simulink model "Controller"  (R2015a)
settings: Solver=ode3  SolverMode=SingleTasking  StartTime=0.0  StopTime=100  FixedStep=T_sim  RelTol=1e-3
PreLoadFcn:
  | LoadLibraries
values from neighbouring files (symbols this model uses):
  a = 10.26    [SetupComplete.m]
  A_x = 0.015    [SetupComplete.m]
  A_y = A_x    (= 0.015)    [SetupComplete.m]
  A_z = 0.16    [SetupComplete.m]
  C_d0 = 0.001193    [SetupComplete.m]
  C_x = 1.2    [SetupComplete.m]
  C_y = C_x    (= 1.2)    [SetupComplete.m]
  C_z = 2.2    [SetupComplete.m]
  CG_0 = [0,0,0.02]'    [SetupComplete.m]
  eta_23 = deg2rad(-1.42)    [Run3Copter.m]
  g = 9.81    [SetupComplete.m]
  h = 0.08    [SetupComplete.m]
  h_M = 0.064    [SetupComplete.m]
  I_BAC_0 = [ Ix,0,Ixz;0,Iy,0;Ixz,0,Iz]    [SetupComplete.m]
  Initial_Omegas = [1;1;1]*Omega_hover    [Run3Copter.m]
  l = 0.3450    (= 0.345)    [NDI_components.m]    (also in SetupComplete.m; robust_controller.m)
  l_arm = 0.264    [SetupComplete.m]
  m = 3.51    [SetupComplete.m]
  m_0 = 2.61    [SetupComplete.m]
  m_M = 0.300    (= 0.3)    [SetupComplete.m]
  R = 0.1778    [SetupComplete.m]    (also in robust_controller.m = eye(4))
  rho = 1.15    [SetupComplete.m]
  sigma = b*c/(pi*R)    (= 0.107416159567)    [SetupComplete.m]
  theta_0 = 0.38397    [SetupComplete.m]
  theta_1 = -0.2967    [SetupComplete.m]
  v_i0 = sqrt( 1/3*m*g/(2*rho*pi*R^2)  )    [SetupComplete.m]
undefined symbols (not defined in the file or in its folder): DOWN_0, EAST_0, Motor, NORTH_0, P_0, Prop, Q_0, R_0, Throttle_Hover, U_0, V_0, v_i_adim, Vx_adim, Vz_adim, W_0
undefined symbols (not defined in the file): Initial_Torques, J_FA, J_T, Rotation_sign, Tau_motors
libraries: XXCopter x39, simulink x35, vrlib x15, simulink_extras x7, aerolib6dofsys x2, qcatlib x2, dspinverses x2
(part 1 of 10)
settings Model: ExtModeTrigDuration=5000  Creator=DavidTorres  LastModifiedBy=juan
settings OptimizationCC: BlockReduction=off  BooleanDataType=off
settings DebuggingCC: SaveWithParameterizedLinksMsg=none  UnderspecifiedInitializationDetection=Classic  MergeDetectMultiDrivingBlocksExec=none
settings HardwareCC: TargetUnknown=on

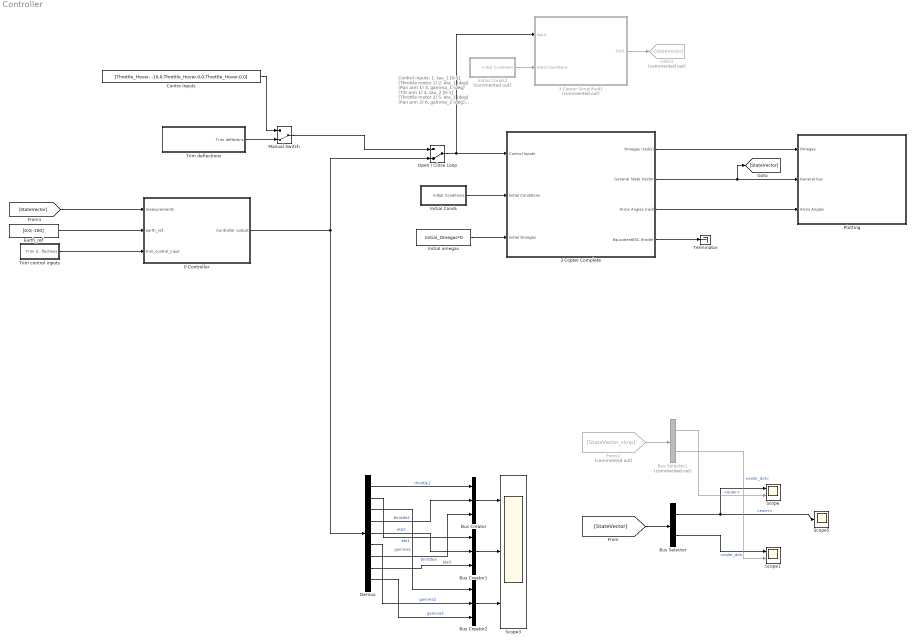
== system Controller ==
  note: Control inputs:
      | 1. tau_1 [0-1] (Throttle motor 1)
      | 2. eta_1 (deg)  (Pan arm 1)
      | 3. gamma_1 (deg)  (Tilt arm 1)
      |
      | 4. tau_2 [0-1] (Throttle motor 2)
      | 5. eta_2 (deg)  (Pan arm 2)
      | 6. gamma_2 (deg)  (Tilt arm 2)
      |
      | 7. tau_3 [0-1] (Throttle motor 3)
      | 8. eta_3 (deg)  (Pan arm  3)
      | 9. gamma_3 (deg)  (Tilt arm 3)
  3 Copter Complete : Subsystem
  3 Copter Simplified1 : Subsystem  Commented=on
  Bus Creator : BusCreator  Inputs=3
  Bus Creator1 : BusCreator  Inputs=3
  Bus Creator2 : BusCreator  Inputs=3
  Bus Selector : BusSelector  OutputSignals=euler,euler_dot
  Bus Selector1 : BusSelector  Commented=on  OutputSignals=euler,euler_dot
  Contro Inputs : Constant  Value=[Throttle_Hover, -10,0,Throttle_Hover,0,0,Throttle_Hover,0,0]
  Demux : Demux  Outputs=9
  Earth_ref : Constant  Value=[0;0;-100]
  From2 : From  Commented=on  GotoTag=StateVector_simp
  Goto1 : Goto  Commented=on  GotoTag=StateVector
  Initial Conds : Subsystem  TreatAsAtomicUnit=on
  Initial Conds2 : Subsystem  Commented=on  TreatAsAtomicUnit=on
  Initial omegas : Constant  Value=Initial_Omegas*0
  Manual Switch : ManualSwitch  CurrentSetting=0
  Open / Close Loop : ManualSwitch  CurrentSetting=0
  P Controller : Subsystem  Variant=on  OverrideUsingVariant=Variant1
  Plotting : Subsystem
  Scope : Scope  NumInputPorts=2
      settings: YMin=-0.5~-1  YMax=0.5~1  SaveName=ScopeData3
  Scope1 : Scope  NumInputPorts=2
      settings: YMin=-5~-5  YMax=5~5  SaveName=ScopeData4
  Scope3 : Scope  NumInputPorts=3
      settings: ShowLegends=on  TimeRange=100  YMin=0~-6~-1  YMax=1~1~1  SaveName=ScopeData6
  Scope5 : Scope
      settings: YMin=-0.002  YMax=0.01  SaveName=ScopeData13
  Terminator : Terminator
  Trim control inputs : Subsystem  TreatAsAtomicUnit=on
  Trim deflections : Subsystem  TreatAsAtomicUnit=on
  wires:
  Initial omegas/1 -> 3 Copter Complete/3(Initial Omegas)
  Initial Conds/1(Initial Conditions) -> 3 Copter Complete/2(Initial Conditions)
  3 Copter Complete/1(Omegas (rad/s)) -> Plotting/1(Omegas)
  3 Copter Complete/3(Arms Angles (rad)) -> Plotting/3(Arms Angles)
  Contro Inputs/1 -> Manual Switch/1
  Trim deflections/1(Trim deflectins) -> Manual Switch/2
  3 Copter Complete/2(General State Vector) -> [StateVector], Plotting/2(General bus)
  Manual Switch/1 -> Open / Close Loop/1
  [StateVector] -> P Controller/1(measurements)
  P Controller/1(Controller output) -> Demux/1, Open / Close Loop/2
  Trim control inputs/1(Trim deflections) -> P Controller/3(trim_control_input)
  Bus Selector/2 -> Scope1/1  "<euler_dot>"
  Bus Selector/1 -> Scope5/1, Scope/1  "<euler>"
  [StateVector] -> Bus Selector/1
  Demux/2 -> Bus Creator1/1  "eta1"
  Bus Creator/1 -> Scope3/1
  Demux/1 -> Bus Creator/1  "throttle1"
  Demux/4 -> Bus Creator/2  "throttle2"
  Demux/7 -> Bus Creator/3  "throttle3"
  Earth_ref/1 -> P Controller/2(earth_ref)
  3 Copter Complete/4(EquivalentESC throtle) -> Terminator/1
  Initial Conds2/1(Initial Conditions) -> 3 Copter Simplified1/2(Initial Conditions)
  3 Copter Simplified1/1(Out1) -> Goto1/1
  Open / Close Loop/1 -> 3 Copter Complete/1(Control Inputs), 3 Copter Simplified1/1(Input)
  Bus Selector1/2 -> Scope1/2  "<euler_dot>"
  Bus Selector1/1 -> Scope/2  "<euler>"
  From2/1 -> Bus Selector1/1
  Bus Creator1/1 -> Scope3/2
  Demux/5 -> Bus Creator1/2  "eta2"
  Demux/8 -> Bus Creator1/3  "eta3"
  Bus Creator2/1 -> Scope3/3
  Demux/3 -> Bus Creator2/1  "gamma1"
  Demux/6 -> Bus Creator2/2  "gamma2"
  Demux/9 -> Bus Creator2/3  "gamma3"

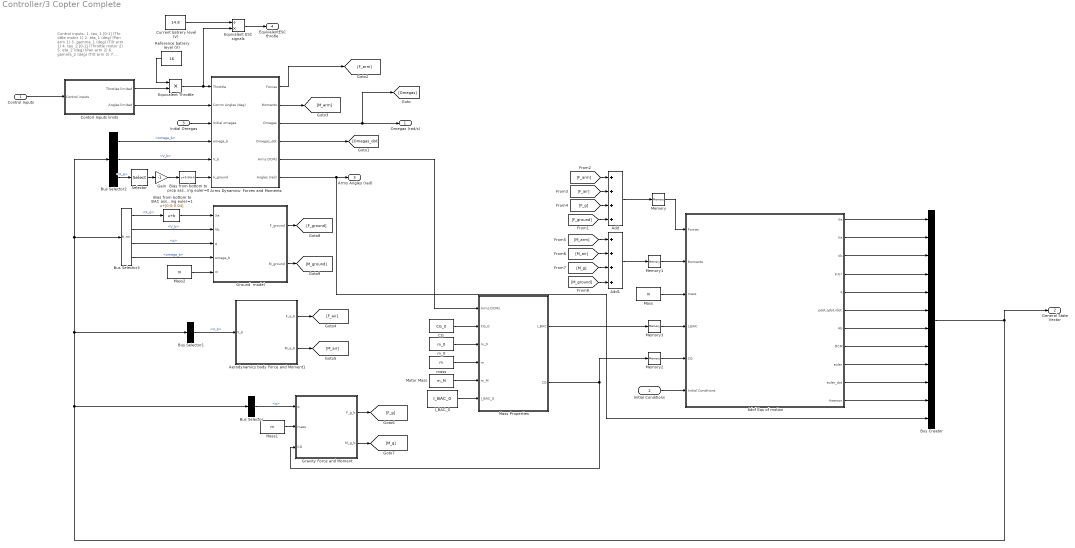
== system Controller/3 Copter Complete ==
  note: Control inputs:
      | 1. tau_1 [0-1] (Thr ottle motor 1)
      | 2. eta_1 (deg)  (Pan arm 1)
      | 3. gamma_1 (deg)  (Tilt arm 1)
      |
      | 4. tau_2 [0-1] (Throttle motor 2)
      | 5. eta_2 (deg)  (Pan arm 2)
      | 6. gamma_2 (deg)  (Tilt arm 2)
      |
      | 7. tau_3 [0-1] (Throttle motor 3)
      | 8. eta_3 (deg)  (Pan arm  3)
      | 9. gamma_3 (deg)  (Tilt arm 3)
  Control Inputs : Inport
  Initial Conditions : Inport  Port=2
  Initial Omegas : Inport  Port=3
  6dof Eqs of motion : Subsystem  TreatAsAtomicUnit=on
  Add : Sum  Inputs=++++
  Add1 : Sum  Inputs=++++
  Aerodynamics body Force and Moment1 : MATLAB Function  TreatAsAtomicUnit=on
  Arms Dynamics: Forces and Moments : Subsystem  Variant=on  OverrideUsingVariant=Variant3
  Bias from bottom to BAC assuming euler=1 : Bias  Bias=[0;0;0.04]
  Bias from bottom to prop assuming euler=0 : Bias  Bias=0.04+h
  Bus Creator : BusCreator  Inputs=12
  Bus Selector : BusSelector  OutputSignals=q
  Bus Selector1 : BusSelector  OutputSignals=V_b
  Bus Selector2 : BusSelector  OutputSignals=omega_b,V_b,X_e
  Bus Selector3 : BusSelector  OutputSignals=X_e,V_b,q,omega_b
  CG : Constant  Value=CG_0
  Contorl Inputs limits : Subsystem  TreatAsAtomicUnit=on
  Current batrery level (V) : Constant  Value=14.8
  Equivalent ESC signals : Product  Inputs=/*
  Equivalent Throttle : Product  Inputs=**
  Gain : Gain  Gain=-1
  Gravity Force and Moment : MATLAB Function  TreatAsAtomicUnit=on
  Ground  model : Subsystem  TreatAsAtomicUnit=on
  I_BAC_0 : Constant  Value=I_BAC_0
  Mass : Constant  Value=m
  Mass Properties : Subsystem  TreatAsAtomicUnit=on
  Mass1 : Constant  Value=m
  Mass2 : Constant  Value=m
  Memory : Memory  X0=[0,0,0]
  Memory1 : Memory  X0=[0,0,0]
  Memory2 : Memory  X0=CG_0
  Memory3 : Memory  X0=I_BAC_0
  Motor Mass : Constant  Value=m_M
  Reference batrery level (V) : Constant  Value=16
  Selector : Selector  InputPortWidth=3  Indices=3
  m_0 : Constant  Value=m_0
  mass : Constant  Value=m
  Omegas (rad/s) : Outport
  General State Vector : Outport  Port=2
  Arms Angles (rad) : Outport  Port=3
  EquivalentESC throtle : Outport  Port=4
  wires:
  Initial Conditions/1 -> 6dof Eqs of motion/6(Initial Conditions)
  6dof Eqs of motion/3(Vb) -> Bus Creator/3
  6dof Eqs of motion/5(q) -> Bus Creator/5
  6dof Eqs of motion/2(Ve) -> Bus Creator/2
  6dof Eqs of motion/6(pdot,qdot,rdot) -> Bus Creator/6
  6dof Eqs of motion/1(Xe) -> Bus Creator/1
  6dof Eqs of motion/7(Ab) -> Bus Creator/7
  6dof Eqs of motion/8(DCM) -> Bus Creator/8
  6dof Eqs of motion/9(euler) -> Bus Creator/9
  6dof Eqs of motion/10(euler_dot) -> Bus Creator/10
  Bus Selector/1 -> Gravity Force and Moment/1(q)  "<q>"
  Mass/1 -> 6dof Eqs of motion/3(mass)
  Mass Properties/1(I_BAC) -> Memory3/1
  Bus Selector1/1 -> Aerodynamics body Force and Moment1/1(V_b)  "<V_b>"
  Bus Selector2/1 -> Arms Dynamics: Forces and Moments/4(omega_b)  "<omega_b>"
  Bus Selector2/2 -> Arms Dynamics: Forces and Moments/5(V_b)  "<V_b>"
  Mass1/1 -> Gravity Force and Moment/2(mass)
  Mass Properties/2(CG) -> Gravity Force and Moment/3(CG), Memory2/1
  Arms Dynamics: Forces and Moments/4(Omegas_dot) -> [Omegas_dot]
  Initial Omegas/1 -> Arms Dynamics: Forces and Moments/3(Initial omegas)
  Bus Selector2/3 -> Selector/1  "<X_e>"
  Selector/1 -> Gain/1
  Gain/1 -> Bias from bottom to prop assuming euler=0/1
  Add/1 -> Memory/1
  Add1/1 -> Memory1/1
  Arms Dynamics: Forces and Moments/1(Forces) -> [F_arm]
  Arms Dynamics: Forces and Moments/2(Moments) -> [M_arm]
  Aerodynamics body Force and Moment1/1(F_a_b) -> [F_air]
  Aerodynamics body Force and Moment1/2(M_a_b) -> [M_air]
  Gravity Force and Moment/1(F_g_b) -> [F_g]
  Gravity Force and Moment/2(M_g_b) -> [M_g]
  [F_arm] -> Add/1
  [F_air] -> Add/2
  [F_g] -> Add/3
  [M_arm] -> Add1/1
  [M_g] -> Add1/3
  [M_air] -> Add1/2
  6dof Eqs of motion/11(Asensor) -> Bus Creator/11
  Contorl Inputs limits/1(Throtles limited) -> Equivalent Throttle/2
  Contorl Inputs limits/2(Angles limited) -> Arms Dynamics: Forces and Moments/2(Comm Angles (deg))
  Arms Dynamics: Forces and Moments/5(Arms DCMs) -> Mass Properties/1(Arms DCMs)
  CG/1 -> Mass Properties/2(CG_0)
  Motor Mass/1 -> Mass Properties/5(m_M)
  I_BAC_0/1 -> Mass Properties/6(I_BAC_0)
  m_0/1 -> Mass Properties/3(m_0)
  mass/1 -> Mass Properties/4(m)
  Arms Dynamics: Forces and Moments/3(Omegas) -> [Omegas], Omegas (rad/s)/1
  Bus Creator/1 -> General State Vector/1, Bus Selector2/1, Bus Selector3/1, Bus Selector1/1, Bus Selector/1
  Memory/1 -> 6dof Eqs of motion/1(Forces)
  Memory1/1 -> 6dof Eqs of motion/2(Moments)
  Memory2/1 -> 6dof Eqs of motion/5(CG)
  Memory3/1 -> 6dof Eqs of motion/4(I_BAC)
  Equivalent Throttle/1 -> Arms Dynamics: Forces and Moments/1(Throttle), Equivalent ESC signals/2
  Reference batrery level (V)/1 -> Equivalent Throttle/1
  Current batrery level (V)/1 -> Equivalent ESC signals/1
  Equivalent ESC signals/1 -> EquivalentESC throtle/1
  6dof Eqs of motion/4(p,q,r) -> Bus Creator/4
  Control Inputs/1 -> Contorl Inputs limits/1(Control inputs)
  Bus Selector3/1 -> Bias from bottom to BAC assuming euler=1/1  "<X_e>"
  Bus Selector3/3 -> Ground  model/3(q)  "<q>"
  Ground  model/1(F_ground) -> [F_ground]
  Ground  model/2(M_ground) -> [M_ground]
  [F_ground] -> Add/4
  [M_ground] -> Add1/4
  Mass2/1 -> Ground  model/5(m)
  Bus Selector3/2 -> Ground  model/2(Vb)  "<V_b>"
  Bus Selector3/4 -> Ground  model/4(omega_b)  "<omega_b>"
  Bias from bottom to prop assuming euler=0/1 -> Arms Dynamics: Forces and Moments/6(h_ground)
  Bias from bottom to BAC assuming euler=1/1 -> Ground  model/1(Xe)
  Arms Dynamics: Forces and Moments/6(Angles (rad)) -> Bus Creator/12, Arms Angles (rad)/1

== system Controller/3 Copter Simplified1 ==
  Input : Inport
  Initial Conditions : Inport  Port=2
  6dof Eqs of motion : Subsystem  TreatAsAtomicUnit=on
  Add : Sum
  Add1 : Sum
  Bus Selector : BusSelector  OutputSignals=V_b,omega_b
  Bus Creator1 : BusCreator  Inputs=11
  Earth to body1 : Product  Multiplication=Matrix(*)
  Gravity : Constant  Value=[0;0;m*g]
  Ground : Ground
  Kq : Constant  Value=0.07
  Kt : Constant  Value=15
  MATLAB Function : MATLAB Function  TreatAsAtomicUnit=on
  Mass : Constant  Value=m
  Mass1 : Constant  Value=|
      | [ 0.1602  0      -0.0080 ;
      |      0       0.2042  0      ;
      |     -0.0080  0       0.3441];
  Mass2 : Constant  Value="[0         0   -0.0015]"
  Memory : Memory  X0=[0,0,0]
  Memory1 : Memory  X0=[0,0,0]
  Permute Dimensions : PermuteDimensions
  Product : Product
  Trimmed actuator signals1 : Display
  deg2rad : Constant  Value=[1, pi/180, pi/180,1, pi/180,pi/180, 1, pi/180,pi/180]
  Out1 : Outport
  wires:
  [gforce_body] -> Add/2
  Memory1/1 -> 6dof Eqs of motion/2(Moments)
  6dof Eqs of motion/2(Ve) -> Bus Creator1/2
  Initial Conditions/1 -> 6dof Eqs of motion/6(Initial Conditions)
  6dof Eqs of motion/11(Asensor) -> Bus Creator1/11
  6dof Eqs of motion/10(euler_dot) -> Bus Creator1/10
  6dof Eqs of motion/4(p,q,r) -> Bus Creator1/4
  MATLAB Function/2(Mbody_ext) -> Add1/1
  6dof Eqs of motion/1(Xe) -> Bus Creator1/1
  Add1/1 -> Memory1/1
  MATLAB Function/1(Tbody_ext) -> Add/1
  6dof Eqs of motion/8(DCM) -> Bus Creator1/8, [DCM]
  Mass/1 -> 6dof Eqs of motion/3(mass)
  6dof Eqs of motion/9(euler) -> Bus Creator1/9
  6dof Eqs of motion/6(pdot,qdot,rdot) -> Bus Creator1/6
  6dof Eqs of motion/7(Ab) -> Bus Creator1/7
  6dof Eqs of motion/3(Vb) -> Bus Creator1/3
  Memory/1 -> 6dof Eqs of motion/1(Forces)
  6dof Eqs of motion/5(q) -> Bus Creator1/5
  Add/1 -> Memory/1
  Ground/1 -> Add1/2
  Mass2/1 -> 6dof Eqs of motion/5(CG)
  Mass1/1 -> 6dof Eqs of motion/4(I_BAC)
  Gravity/1 -> Earth to body1/2
  Earth to body1/1 -> Trimmed actuator signals1/1, [gforce_body]
  [DCM] -> Permute Dimensions/1
  Permute Dimensions/1 -> Earth to body1/1
  Product/1 -> MATLAB Function/1(input)
  deg2rad/1 -> Product/2
  Input/1 -> Product/1
  Kt/1 -> MATLAB Function/2(Kt)
  Kq/1 -> MATLAB Function/3(Kq)
  Bus Creator1/1 -> Bus Selector/1, Out1/1
  Bus Selector/1 -> MATLAB Function/4(v_body)  "<V_b>"
  Bus Selector/2 -> MATLAB Function/5(omega_body)  "<omega_b>"

== system Controller/Initial Conds ==
  Bus Creator : BusCreator
  Ini Position X_e_0 : Constant  Value=[0;0;-100]
  Initial Attitude Euler_0 : Constant  Value=[deg2rad(0);deg2rad(0);deg2rad(0)]
  Initial Attitude Rate  Euler_dot_0 : Constant  Value=[deg2rad(0);deg2rad(0);deg2rad(0)]
  Initial Velocity V_e_0 : Constant  Value=[0;0;0]
  Initial Conditions : Outport
  wires:
  Ini Position X_e_0/1 -> Bus Creator/1  "X_e_0"
  Initial Velocity V_e_0/1 -> Bus Creator/2  "V_e_0"
  Initial Attitude Euler_0/1 -> Bus Creator/3  "Euler_0"
  Initial Attitude Rate  Euler_dot_0/1 -> Bus Creator/4  "Euler_dot_0"
  Bus Creator/1 -> Initial Conditions/1

== system Controller/Initial Conds2 ==
  Bus Creator : BusCreator
  Ini Position X_e_0 : Constant  Value=[0;0;-100]
  Initial Attitude Euler_0 : Constant  Value=[deg2rad(0);deg2rad(0);deg2rad(0)]
  Initial Attitude Rate  Euler_dot_0 : Constant  Value=[deg2rad(0);deg2rad(0);deg2rad(0)]
  Initial Velocity V_e_0 : Constant  Value=[0;0;0]
  Initial Conditions : Outport
  wires:
  Bus Creator/1 -> Initial Conditions/1
  Initial Attitude Rate  Euler_dot_0/1 -> Bus Creator/4  "Euler_dot_0"
  Initial Attitude Euler_0/1 -> Bus Creator/3  "Euler_0"
  Initial Velocity V_e_0/1 -> Bus Creator/2  "V_e_0"
  Ini Position X_e_0/1 -> Bus Creator/1  "X_e_0"

== system Controller/P Controller ==
  note: Controller output:
      | Throttle [%]
      | Actuator angle [deg]
  note: Controller output:
      | 1. tau_1 [0-1] (Thr ottle motor 1)
      | 2. eta_1 (deg)  (Pan arm 1)
      | 3. gamma_1 (deg)  (Tilt arm 1)
      |
      | 4. tau_2 [0-1] (Throttle motor 2)
      | 5. eta_2 (deg)  (Pan arm 2)
      | 6. gamma_2 (deg)  (Tilt arm 2)
      |
      | 7. tau_3 [0-1] (Throttle motor 3)
      | 8. eta_3 (deg)  (Pan arm  3)
      | 9. gamma_3 (deg)  (Tilt arm 3)
  measurements : Inport
  earth_ref : Inport  Port=2
  trim_control_input : Inport  Port=3
  4DOF PID Controller : Subsystem  Variant=on  VariantControl=(default)  OverrideUsingVariant=Variant3
  NDI+CA Controller : Subsystem  Variant=on  VariantControl=Variant1  OverrideUsingVariant=Variant1
  Controller output : Outport

== system Controller/Plotting ==
  Omegas : Inport
  General bus : Inport  Port=2
  Arms Angles : Inport  Port=3
  Bus Creator : BusCreator  Inputs=3
  Bus Selector : BusSelector  OutputSignals=euler,X_e,DCM
  Bus Selector1 : BusSelector  OutputSignals=Angles Arm 1,Angles Arm 2,Angles Arm 3
  Demux : Demux  Outputs=3
  Gain : Gain  Gain=180/pi
  Level-2 MATLAB S-Function : M-S-Function  Commented=on  FunctionName=Simulation_3_copter
  Scope : Scope  NumInputPorts=2
      settings: ShowLegends=on  YMin=-5~-200  YMax=15~100
  Scope1 : Scope
      settings: TimeRange=5  YMin=672.75  YMax=676.75
  Scope2 : Scope  NumInputPorts=3
      settings: ShowLegends=on  YMin=-0.045~-1~-1  YMax=0~1~1  SaveName=ScopeData2
  wires:
  General bus/1 -> Bus Selector/1
  Omegas/1 -> Scope1/1  "Omegas"
  Arms Angles/1 -> Bus Selector1/1
  Bus Selector1/3 -> Scope2/3, Level-2 MATLAB S-Function/8  "<Angles Arm 3>"
  Bus Selector1/2 -> Level-2 MATLAB S-Function/7, Scope2/2  "<Angles Arm 2>"
  Bus Selector1/1 -> Level-2 MATLAB S-Function/6, Scope2/1  "<Angles Arm 1>"
  Bus Selector/2 -> Level-2 MATLAB S-Function/1, Scope/2  "<X_e>"
  [r_p_3] -> Level-2 MATLAB S-Function/5
  [r_p_2] -> Level-2 MATLAB S-Function/4
  [r_p_1] -> Level-2 MATLAB S-Function/3
  Bus Selector/3 -> Level-2 MATLAB S-Function/2  "<DCM>"
  Demux/3 -> Bus Creator/3  "psi(deg)"
  Demux/1 -> Bus Creator/1  "phi(deg)"
  Demux/2 -> Bus Creator/2  "theta(deg)"
  Bus Creator/1 -> Scope/1
  Bus Selector/1 -> Gain/1  "<euler>"
  Gain/1 -> Demux/1

== system Controller/Trim control inputs ==
  Contro Inputs1 : Constant  Value=0.59
  Contro Inputs2 : Constant  Value=0.5889
  Contro Inputs3 : Constant  Value=0.5896
  Contro Inputs4 : Constant  Value=-2.298
  Ground : Ground
  Mux : Mux  Inputs=9
  Trim deflections : Outport
  wires:
  Mux/1 -> Trim deflections/1
  Ground/1 -> Mux/3, Mux/5, Mux/8, Mux/9, Mux/6
  Contro Inputs2/1 -> Mux/4
  Contro Inputs1/1 -> Mux/1
  Contro Inputs4/1 -> Mux/2
  Contro Inputs3/1 -> Mux/7

== system Controller/Trim deflections ==
  " " : simulink_extras/Transformations/Radians to Degrees
  Contro Inputs1 : Constant  Value=Throttle_Hover
  Contro Inputs2 : Constant  Value=Throttle_Hover
  Contro Inputs3 : Constant  Value=eta_23
  Gain : Gain  Gain=-1
  Ground : Ground
  Mux : Mux  Inputs=9
  Trim deflectins : Outport
  wires:
  Contro Inputs1/1 -> Mux/1
  Contro Inputs2/1 -> Mux/7, Mux/4
  Ground/1 -> Mux/2, Mux/6, Mux/9, Mux/3
  Contro Inputs3/1 -> " "/1
  " "/1 -> Gain/1, Mux/5
  Gain/1 -> Mux/8
  Mux/1 -> Trim deflectins/1

== system Controller/3 Copter Complete/6dof Eqs of motion ==
  Forces : Inport
  Moments : Inport  Port=2
  mass : Inport  Port=3
  I_BAC : Inport  Port=4
  CG : Inport  Port=5
  Initial Conditions : Inport  Port=6
  Accelerometer meas : MATLAB Function  TreatAsAtomicUnit=on
  Bus Selector : BusSelector  OutputSignals=X_e_0,V_e_0,Euler_0,Euler_dot_0
  DCM1 : Subsystem  TreatAsAtomicUnit=on
  Normalize 4D vector : Subsystem  AncestorBlock=XXCopter/Normalize 4D vector  TreatAsAtomicUnit=on
  Position Eqs : MATLAB Function  TreatAsAtomicUnit=on
  Rotational eqs : MATLAB Function  TreatAsAtomicUnit=on
  SVFI_to_SVFb : MATLAB Function  TreatAsAtomicUnit=on
  SV_F_b_to_SV_FI : MATLAB Function  TreatAsAtomicUnit=on
  Selector7 : Selector  InputPortWidth=3  Indices=[3 2 1]
  "p,q,r " : Integrator  InitialConditionSource=external  InitialCondition=[P_0,Q_0,R_0]
  q_dot : Subsystem  TreatAsAtomicUnit=on
  quaternion : Integrator  InitialConditionSource=external  InitialCondition=[P_0,Q_0,R_0]
  ub,vb,wb : Integrator  InitialConditionSource=external  InitialCondition=[U_0,V_0,W_0]
  xe,ye,ze : Integrator  InitialConditionSource=external  InitialCondition=[NORTH_0,EAST_0,-DOWN_0]
  Xe : Outport
  Ve : Outport  Port=2
  Vb : Outport  Port=3
  p,q,r : Outport  Port=4
  q : Outport  Port=5
  pdot,qdot,rdot : Outport  Port=6
  Ab : Outport  Port=7
  DCM : Outport  Port=8
  euler : Outport  Port=9
  euler_dot : Outport  Port=10
  Asensor : Outport  Port=11
  wires:
  I_BAC/1 -> Rotational eqs/3(I_BAC)
  mass/1 -> Position Eqs/5(m)
  Forces/1 -> Position Eqs/4(Forces)
  xe,ye,ze/1 -> Xe/1  "X_e"
  ub,vb,wb/1 -> Vb/1, Accelerometer meas/1(Vb), Position Eqs/1(Vb), SV_F_b_to_SV_FI/1(V_b)  "V_b"
  SV_F_b_to_SV_FI/1(V_e) -> Ve/1, xe,ye,ze/1  "V_e"
  [omega] -> Position Eqs/2(omega)
  [omega_dot] -> Position Eqs/3(omega_dot)
  Position Eqs/1(A_b) -> ub,vb,wb/1, Ab/1, Accelerometer meas/4(Ab)  "A_b"
  CG/1 -> Position Eqs/6(CG)
  Initial Conditions/1 -> Bus Selector/1
  Bus Selector/1 -> SVFI_to_SVFb/1(X_e)  "<X_e_0>"
  Bus Selector/2 -> SVFI_to_SVFb/2(V_e)  "<V_e_0>"
  Bus Selector/3 -> SVFI_to_SVFb/3(Euler_Ang)  "<Euler_0>"
  Bus Selector/4 -> SVFI_to_SVFb/4(Euler_Ang_Dot)  "<Euler_dot_0>"
  SVFI_to_SVFb/2(V_b) -> ub,vb,wb/2
  SVFI_to_SVFb/1(X_e_out) -> xe,ye,ze/2
  SVFI_to_SVFb/3(omega_b) -> "p,q,r "/2
  Rotational eqs/1(omega_dot) -> pdot,qdot,rdot/1, [omega_dot], "p,q,r "/1
  "p,q,r "/1 -> q_dot/1(omega_b), [omega], p,q,r/1, Rotational eqs/1(omega_b)  "omega_b"
  q_dot/1(q_dot) -> quaternion/1, SV_F_b_to_SV_FI/2(q_dot)
  SVFI_to_SVFb/4(q) -> quaternion/2
  quaternion/1 -> Normalize 4D vector/1(v), q_dot/2(q)  "q"
  SV_F_b_to_SV_FI/2(euler) -> Selector7/1, euler/1  "euler"
  SV_F_b_to_SV_FI/3(euler_dot) -> euler_dot/1  "euler_dot"
  Moments/1 -> Rotational eqs/2(Moments)
  Normalize 4D vector/1(normal(v)) -> q/1, SV_F_b_to_SV_FI/3(q)  "q"
  [omega] -> Accelerometer meas/2(omega)
  [omega_dot] -> Accelerometer meas/3(omega_dot)
  Accelerometer meas/1(A_s) -> Asensor/1
  DCM1/1(DCM) -> DCM/1  "DCM"
  Selector7/1 -> DCM1/1(Euler)

== system Controller/3 Copter Complete/Arms Dynamics: Forces and Moments ==
  note: 1) Add Subsystem or Model blocks as valid variant choices.
      | 2) You cannot connect blocks at this level. At simulation, connectivity is automatically
      | determined, based on the active variant and port name matching.
  Throttle : Inport
  Comm Angles (deg) : Inport  Port=2
  Initial omegas : Inport  Port=3
  omega_b : Inport  Port=4
  V_b : Inport  Port=5
  h_ground : Inport  Port=6
  4 DOF Arms Dynamics: Forces and Moments1 : Subsystem  VariantControl=Variant3
  9 DOF Arms Dynamics: Forces and Moments : Subsystem  VariantControl=Variant2
  Forces : Outport
  Moments : Outport  Port=2
  Omegas : Outport  Port=3
  Omegas_dot : Outport  Port=4
  Arms DCMs : Outport  Port=5
  Angles (rad) : Outport  Port=6

== system Controller/3 Copter Complete/Contorl Inputs limits ==
  note: limits in degs
  Control inputs : Inport
  Demux : Demux  Outputs=6
  Mux : Mux  Inputs=6
  Saturation : Saturate  UpperLimit=1  LowerLimit=0  LinearizeAsGain=off
  Throttles : Selector  InputPortWidth=9  Indices=[1,4,7]
  "angles " : Selector  InputPortWidth=9  Indices=[2,3,5,6,8,9]
  eta 1 : Saturate  UpperLimit=180  LowerLimit=-180
  eta 2 : Saturate  UpperLimit=180  LowerLimit=-180
  eta 3 : Saturate  UpperLimit=180  LowerLimit=-180
  gamma 2 : Saturate  UpperLimit=90  LowerLimit=-30
  gamma1 : Saturate  UpperLimit=30  LowerLimit=-90
  gamma3 : Saturate  UpperLimit=30  LowerLimit=-90
  Throtles limited : Outport
  Angles limited : Outport  Port=2
  wires:
  Control inputs/1 -> Throttles/1, "angles "/1
  Throttles/1 -> Saturation/1
  "angles "/1 -> Demux/1
  Demux/1 -> eta 1/1
  Demux/2 -> gamma1/1
  Demux/3 -> eta 2/1
  Demux/4 -> gamma 2/1
  Demux/5 -> eta 3/1
  Demux/6 -> gamma3/1
  eta 1/1 -> Mux/1
  gamma1/1 -> Mux/2
  eta 2/1 -> Mux/3
  gamma 2/1 -> Mux/4
  eta 3/1 -> Mux/5
  gamma3/1 -> Mux/6
  Mux/1 -> Angles limited/1
  Saturation/1 -> Throtles limited/1

== system Controller/3 Copter Complete/Ground  model ==
  Xe : Inport
  Vb : Inport  Port=2
  q : Inport  Port=3
  omega_b : Inport  Port=4
  m : Inport  Port=5
  Ground model logic and Forces and moments : MATLAB Function  TreatAsAtomicUnit=on
  arm_hub position 1 : Constant  Value=l*[1;0;0]
  arm_hub position 2 : Constant  Value=l*[-1/2;sqrt(3)/2;0]
  arm_hub position 3 : Constant  Value=l*[-1/2;-sqrt(3)/2;0]
  F_ground : Outport
  M_ground : Outport  Port=2
  wires:
  Xe/1 -> Ground model logic and Forces and moments/1(Xe)
  q/1 -> Ground model logic and Forces and moments/3(q)
  m/1 -> Ground model logic and Forces and moments/5(mass)
  arm_hub position 1/1 -> Ground model logic and Forces and moments/6(Arm1)
  arm_hub position 2/1 -> Ground model logic and Forces and moments/7(Arm2)
  arm_hub position 3/1 -> Ground model logic and Forces and moments/8(Arm3)
  Ground model logic and Forces and moments/2(M_gr_b) -> M_ground/1
  Ground model logic and Forces and moments/1(F_gr_b) -> F_ground/1
  Vb/1 -> Ground model logic and Forces and moments/2(Vb)
  omega_b/1 -> Ground model logic and Forces and moments/4(omega_b)

== system Controller/3 Copter Complete/Mass Properties ==
  Arms DCMs : Inport
  CG_0 : Inport  Port=2
  m_0 : Inport  Port=3
  m : Inport  Port=4
  m_M : Inport  Port=5
  I_BAC_0 : Inport  Port=6
  Arm Inertia : MATLAB Function  TreatAsAtomicUnit=on
  Bus Selector : BusSelector  OutputSignals=T_FaFb1,T_FaFb2,T_FaFb3
  CG position : Sum
  Divide : Product  Inputs=*/
  Divide1 : Product  Inputs=**
  Divide2 : Product  Inputs=/*
  Divide3 : Product  Inputs=**
  Motors Pos sum : Sum  Inputs=+++
  Total I_BAC : Sum
  I_BAC : Outport
  CG : Outport  Port=2
  wires:
  Arms DCMs/1 -> Bus Selector/1
  Bus Selector/3 -> Arm Inertia/3(T3_FAFb)  "<T_FaFb3>"
  Bus Selector/2 -> Arm Inertia/2(T2_FAFb)  "<T_FaFb2>"
  Bus Selector/1 -> Arm Inertia/1(T1_FAFb)  "<T_FaFb1>"
  Total I_BAC/1 -> I_BAC/1
  m_0/1 -> Divide/1
  m/1 -> Divide/2, Divide2/1
  CG_0/1 -> Divide1/1
  Divide/1 -> Divide1/2
  m_M/1 -> Divide2/2
  CG position/1 -> CG/1
  Divide1/1 -> CG position/1
  Motors Pos sum/1 -> Divide3/1
  Divide2/1 -> Divide3/2
  Divide3/1 -> CG position/2
  Arm Inertia/3(r2_M) -> Motors Pos sum/2
  Arm Inertia/4(r3_M) -> Motors Pos sum/1
  Arm Inertia/1(I_M) -> Total I_BAC/2
  I_BAC_0/1 -> Total I_BAC/1
  Arm Inertia/2(r1_M) -> Motors Pos sum/3

== system Controller/3 Copter Simplified1/6dof Eqs of motion ==
  note: This is T_Fb->Fe
  Forces : Inport
  Moments : Inport  Port=2
  mass : Inport  Port=3
  I_BAC : Inport  Port=4
  CG : Inport  Port=5
  Initial Conditions : Inport  Port=6
  Accelerometer meas : MATLAB Function  TreatAsAtomicUnit=on
  Bus Selector : BusSelector  OutputSignals=X_e_0,V_e_0,Euler_0,Euler_dot_0
  DCM1 : Subsystem  TreatAsAtomicUnit=on
  Normalize 4D vector : Subsystem  AncestorBlock=XXCopter/Normalize 4D vector  TreatAsAtomicUnit=on
  Position Eqs : MATLAB Function  TreatAsAtomicUnit=on
  Rotational eqs : MATLAB Function  TreatAsAtomicUnit=on
  SVFI_to_SVFb : MATLAB Function  TreatAsAtomicUnit=on
  SV_F_b_to_SV_FI : MATLAB Function  TreatAsAtomicUnit=on
  Selector7 : Selector  InputPortWidth=3  Indices=[3 2 1]
  "p,q,r " : Integrator  InitialConditionSource=external  InitialCondition=[P_0,Q_0,R_0]
  q_dot : Subsystem  TreatAsAtomicUnit=on
  quaternion : Integrator  InitialConditionSource=external  InitialCondition=[P_0,Q_0,R_0]
  ub,vb,wb : Integrator  InitialConditionSource=external  InitialCondition=[U_0,V_0,W_0]
  xe,ye,ze : Integrator  InitialConditionSource=external  InitialCondition=[NORTH_0,EAST_0,-DOWN_0]
  Xe : Outport
  Ve : Outport  Port=2
  Vb : Outport  Port=3
  p,q,r : Outport  Port=4
  q : Outport  Port=5
  pdot,qdot,rdot : Outport  Port=6
  Ab : Outport  Port=7
  DCM : Outport  Port=8
  euler : Outport  Port=9
  euler_dot : Outport  Port=10
  Asensor : Outport  Port=11
  wires:
  I_BAC/1 -> Rotational eqs/3(I_BAC)
  mass/1 -> Position Eqs/5(m)
  Forces/1 -> Position Eqs/4(Forces)
  xe,ye,ze/1 -> Xe/1  "X_e"
  ub,vb,wb/1 -> Vb/1, Accelerometer meas/1(Vb), Position Eqs/1(Vb), SV_F_b_to_SV_FI/1(V_b)  "V_b"
  SV_F_b_to_SV_FI/1(V_e) -> Ve/1, xe,ye,ze/1  "V_e"
  [omega] -> Position Eqs/2(omega)
  [omega_dot] -> Position Eqs/3(omega_dot)
  Position Eqs/1(A_b) -> ub,vb,wb/1, Ab/1, Accelerometer meas/4(Ab)  "A_b"
  CG/1 -> Position Eqs/6(CG)
  Initial Conditions/1 -> Bus Selector/1
  Bus Selector/1 -> SVFI_to_SVFb/1(X_e)  "<X_e_0>"
  Bus Selector/2 -> SVFI_to_SVFb/2(V_e)  "<V_e_0>"
  Bus Selector/3 -> SVFI_to_SVFb/3(Euler_Ang)  "<Euler_0>"
  Bus Selector/4 -> SVFI_to_SVFb/4(Euler_Ang_Dot)  "<Euler_dot_0>"
  SVFI_to_SVFb/2(V_b) -> ub,vb,wb/2
  SVFI_to_SVFb/1(X_e_out) -> xe,ye,ze/2
  SVFI_to_SVFb/3(omega_b) -> "p,q,r "/2
  Rotational eqs/1(omega_dot) -> pdot,qdot,rdot/1, [omega_dot], "p,q,r "/1
  "p,q,r "/1 -> q_dot/1(omega_b), [omega], p,q,r/1, Rotational eqs/1(omega_b)  "omega_b"
  q_dot/1(q_dot) -> quaternion/1, SV_F_b_to_SV_FI/2(q_dot)
  SVFI_to_SVFb/4(q) -> quaternion/2
  quaternion/1 -> Normalize 4D vector/1(v), q_dot/2(q)  "q"
  SV_F_b_to_SV_FI/2(euler) -> Selector7/1, euler/1  "euler"
  SV_F_b_to_SV_FI/3(euler_dot) -> euler_dot/1  "euler_dot"
  Moments/1 -> Rotational eqs/2(Moments)
  Normalize 4D vector/1(normal(v)) -> q/1, SV_F_b_to_SV_FI/3(q)  "q"
  [omega] -> Accelerometer meas/2(omega)
  [omega_dot] -> Accelerometer meas/3(omega_dot)
  Accelerometer meas/1(A_s) -> Asensor/1
  DCM1/1(DCM) -> DCM/1  "DCM"
  Selector7/1 -> DCM1/1(Euler)

== system Controller/P Controller/4DOF PID Controller ==
  measurements : Inport
  earth_ref : Inport  Port=2
  trim_control_input : Inport  Port=3
  4DOF PI Angle Controller : Subsystem  VariantControl=Variant1
  4DOF PI Angle Trimming Controller : Subsystem  VariantControl=Variant4
  4DOF PI Rate Trimming Controller : Subsystem  VariantControl=Variant2
  4DOF PID Speed Controller : Subsystem  VariantControl=Variant3
  Controller output : Outport

== system Controller/P Controller/NDI+CA Controller ==
  measurements : Inport
  earth_ref : Inport  Port=2
  trim_control_input : Inport  Port=3
  " 9DOF NDI+CA Controller - No massic update" : Subsystem  VariantControl=Variant2
  4DOF NDI+CA Controller : Subsystem  VariantControl=Variant3
  4DOF NDI+CA Controller - No massic update : Subsystem  VariantControl=Variant1
  9DOF NDI+CA Controller : Subsystem  VariantControl=(default)
  Controller output : Outport

== system Controller/3 Copter Complete/6dof Eqs of motion/DCM1 ==
  Euler : Inport  PortDimensions=3
  Fcn11 : Fcn  Expr=u(5)*u(4)
  Fcn12 : Fcn  Expr=u(5)*u(1)
  Fcn13 : Fcn  Expr=-u(2)
  Fcn21 : Fcn  Expr=u(3)*u(2)*u(4) - u(6)*u(1)
  Fcn22 : Fcn  Expr=u(3)*u(2)*u(1) + u(6)*u(4)
  Fcn23 : Fcn  Expr=u(3)*u(5)
  Fcn31 : Fcn  Expr=u(6)*u(2)*u(4) + u(3)*u(1)
  Fcn32 : Fcn  Expr=u(6)*u(2)*u(1) - u(3)*u(4)
  Fcn33 : Fcn  Expr=u(6)*u(5)
  Mux : Mux  Inputs=2
  Mux1 : Mux  Inputs=9
  Reshape : Reshape  OutputDimensionality=Customize  OutputDimensions=[3,3]
  sincos : Trigonometry  Operator=sincos
  DCM : Outport  PortDimensions=[3,3]
  wires:
  Fcn33/1 -> Mux1/9
  Fcn32/1 -> Mux1/8
  Fcn23/1 -> Mux1/6
  Fcn22/1 -> Mux1/5
  Fcn31/1 -> Mux1/7
  Fcn21/1 -> Mux1/4
  Fcn13/1 -> Mux1/3
  Fcn12/1 -> Mux1/2
  Fcn11/1 -> Mux1/1
  Mux/1 -> Fcn22/1, Fcn23/1, Fcn31/1, Fcn33/1, Fcn32/1, Fcn21/1, Fcn13/1, Fcn12/1, Fcn11/1
  sincos/2 -> Mux/2
  sincos/1 -> Mux/1
  Reshape/1 -> DCM/1
  Euler/1 -> sincos/1
  Mux1/1 -> Reshape/1

== system Controller/3 Copter Complete/6dof Eqs of motion/Normalize 4D vector ==
  v : Inport
  4D vec norm : XXCopter/4D vec norm
  Bias : Bias  Bias=eps
  Demux : Demux
  Math Function : Math  Operator=reciprocal  SaturateOnIntegerOverflow=on
  Mux : Mux
  Product{1..4} (4 alike) : Product  Inputs=**
  normal(v) : Outport
  wires:
  Bias/1 -> Math Function/1
  Product1/1 -> Mux/3
  Math Function/1 -> Product4/2, Product1/2, Product3/2, Product2/2
  Demux/3 -> Product1/1
  Product3/1 -> Mux/2
  Product2/1 -> Mux/1
  4D vec norm/1 -> Bias/1
  v/1 -> 4D vec norm/1, Demux/1
  Mux/1 -> normal(v)/1
  Demux/1 -> Product2/1
  Demux/2 -> Product3/1
  Demux/4 -> Product4/1
  Product4/1 -> Mux/4

== system Controller/3 Copter Complete/6dof Eqs of motion/q_dot ==
  note: Both of these methods to compute q_dot are very similar
  omega_b : Inport
  q : Inport  Port=2
  Quaternion_dot : MATLAB Function  Commented=on  TreatAsAtomicUnit=on  VariantControl=Variant
  chose which method : ManualSwitch
  qdot : aerolib6dofsys/DCM & Euler Angles (Quaternion)/qdot
  q_dot : Outport
  wires:
  omega_b/1 -> Quaternion_dot/1(omega_b), qdot/1  "omega_b"
  q/1 -> Quaternion_dot/2(q), qdot/2  "q"
  chose which method/1 -> q_dot/1
  qdot/1 -> chose which method/1
  Quaternion_dot/1(q_dot) -> chose which method/2

== system Controller/3 Copter Complete/Arms Dynamics: Forces and Moments/4 DOF Arms Dynamics: Forces and Moments1 ==
  Throttle : Inport
  Comm Angles (deg) : Inport  Port=2
  Initial omegas : Inport  Port=3
  omega_b : Inport  Port=4
  V_b : Inport  Port=5
  h_ground : Inport  Port=6
  4 DOF Arms Dynamics: Forces and Moments1 : Subsystem  VariantControl=Variant1
  Forces : Outport
  Moments : Outport  Port=2
  Omegas : Outport  Port=3
  Omegas_dot : Outport  Port=4
  Arms DCMs : Outport  Port=5
  Angles (rad) : Outport  Port=6
  wires:
  Comm Angles (deg)/1 -> 4 DOF Arms Dynamics: Forces and Moments1/2(Comm Angles (deg))
  Initial omegas/1 -> 4 DOF Arms Dynamics: Forces and Moments1/3(Initial Omegas)
  Throttle/1 -> 4 DOF Arms Dynamics: Forces and Moments1/1(Throttles)
  omega_b/1 -> 4 DOF Arms Dynamics: Forces and Moments1/4(omega_b)
  V_b/1 -> 4 DOF Arms Dynamics: Forces and Moments1/5(V_b)
  h_ground/1 -> 4 DOF Arms Dynamics: Forces and Moments1/6(h_ground)
  4 DOF Arms Dynamics: Forces and Moments1/1(Forces) -> Forces/1
  4 DOF Arms Dynamics: Forces and Moments1/2(Moments) -> Moments/1
  4 DOF Arms Dynamics: Forces and Moments1/3(Omegas) -> Omegas/1
  4 DOF Arms Dynamics: Forces and Moments1/4(Omegas_dot) -> Omegas_dot/1
  4 DOF Arms Dynamics: Forces and Moments1/5(Arms DCMs) -> Arms DCMs/1
  4 DOF Arms Dynamics: Forces and Moments1/6(Angles (rad)) -> Angles (rad)/1

== system Controller/3 Copter Complete/Arms Dynamics: Forces and Moments/9 DOF Arms Dynamics: Forces and Moments ==
  Throttle : Inport
  Comm Angles (deg) : Inport  Port=2
  Initial omegas : Inport  Port=3
  omega_b : Inport  Port=4
  V_b : Inport  Port=5
  h_ground : Inport  Port=6
  9 DOF Arms Dynamics: Forces and Moments : Subsystem  VariantControl=Variant
  Forces : Outport
  Moments : Outport  Port=2
  Omegas : Outport  Port=3
  Omegas_dot : Outport  Port=4
  Arms DCMs : Outport  Port=5
  Angles (rad) : Outport  Port=6
  wires:
  h_ground/1 -> 9 DOF Arms Dynamics: Forces and Moments/6(h_ground)
  omega_b/1 -> 9 DOF Arms Dynamics: Forces and Moments/4(omega_b)
  Throttle/1 -> 9 DOF Arms Dynamics: Forces and Moments/1(Throttles)
  Comm Angles (deg)/1 -> 9 DOF Arms Dynamics: Forces and Moments/2(Comm Angles (deg))
  V_b/1 -> 9 DOF Arms Dynamics: Forces and Moments/5(V_b)
  Initial omegas/1 -> 9 DOF Arms Dynamics: Forces and Moments/3(Initial Omegas)
  9 DOF Arms Dynamics: Forces and Moments/1(Forces) -> Forces/1
  9 DOF Arms Dynamics: Forces and Moments/2(Moments) -> Moments/1
  9 DOF Arms Dynamics: Forces and Moments/3(Omegas) -> Omegas/1
  9 DOF Arms Dynamics: Forces and Moments/4(Omegas_dot) -> Omegas_dot/1
  9 DOF Arms Dynamics: Forces and Moments/5(Arms DCMs) -> Arms DCMs/1
  9 DOF Arms Dynamics: Forces and Moments/6(Angles (rad)) -> Angles (rad)/1

== system Controller/3 Copter Simplified1/6dof Eqs of motion/DCM1 ==
  Euler : Inport  PortDimensions=3
  Fcn11 : Fcn  Expr=u(5)*u(4)
  Fcn12 : Fcn  Expr=u(5)*u(1)
  Fcn13 : Fcn  Expr=-u(2)
  Fcn21 : Fcn  Expr=u(3)*u(2)*u(4) - u(6)*u(1)
  Fcn22 : Fcn  Expr=u(3)*u(2)*u(1) + u(6)*u(4)
  Fcn23 : Fcn  Expr=u(3)*u(5)
  Fcn31 : Fcn  Expr=u(6)*u(2)*u(4) + u(3)*u(1)
  Fcn32 : Fcn  Expr=u(6)*u(2)*u(1) - u(3)*u(4)
  Fcn33 : Fcn  Expr=u(6)*u(5)
  Mux : Mux  Inputs=2
  Mux1 : Mux  Inputs=9
  Reshape : Reshape  OutputDimensionality=Customize  OutputDimensions=[3,3]
  sincos : Trigonometry  Operator=sincos
  DCM : Outport  PortDimensions=[3,3]
  wires:
  Fcn33/1 -> Mux1/9
  Fcn32/1 -> Mux1/8
  Fcn23/1 -> Mux1/6
  Fcn22/1 -> Mux1/5
  Fcn31/1 -> Mux1/7
  Fcn21/1 -> Mux1/4
  Fcn13/1 -> Mux1/3
  Fcn12/1 -> Mux1/2
  Fcn11/1 -> Mux1/1
  Mux/1 -> Fcn22/1, Fcn23/1, Fcn31/1, Fcn33/1, Fcn32/1, Fcn21/1, Fcn13/1, Fcn12/1, Fcn11/1
  sincos/2 -> Mux/2
  sincos/1 -> Mux/1
  Reshape/1 -> DCM/1
  Euler/1 -> sincos/1
  Mux1/1 -> Reshape/1

== system Controller/3 Copter Simplified1/6dof Eqs of motion/Normalize 4D vector ==
  v : Inport
  4D vec norm : XXCopter/4D vec norm
  Bias : Bias  Bias=eps
  Demux : Demux
  Math Function : Math  Operator=reciprocal  SaturateOnIntegerOverflow=on
  Mux : Mux
  Product{1..4} (4 alike) : Product  Inputs=**
  normal(v) : Outport
  wires:
  Bias/1 -> Math Function/1
  Product1/1 -> Mux/3
  Math Function/1 -> Product4/2, Product1/2, Product3/2, Product2/2
  Demux/3 -> Product1/1
  Product3/1 -> Mux/2
  Product2/1 -> Mux/1
  4D vec norm/1 -> Bias/1
  v/1 -> 4D vec norm/1, Demux/1
  Mux/1 -> normal(v)/1
  Demux/1 -> Product2/1
  Demux/2 -> Product3/1
  Demux/4 -> Product4/1
  Product4/1 -> Mux/4

== system Controller/3 Copter Simplified1/6dof Eqs of motion/q_dot ==
  note: Both of these methods to compute q_dot are very similar
  omega_b : Inport
  q : Inport  Port=2
  Quaternion_dot : MATLAB Function  TreatAsAtomicUnit=on  VariantControl=Variant
  chose which method : ManualSwitch  CurrentSetting=0
  qdot : aerolib6dofsys/DCM & Euler Angles (Quaternion)/qdot  Commented=on
  q_dot : Outport
  wires:
  omega_b/1 -> Quaternion_dot/1(omega_b), qdot/1  "omega_b"
  q/1 -> Quaternion_dot/2(q), qdot/2  "q"
  chose which method/1 -> q_dot/1
  qdot/1 -> chose which method/1
  Quaternion_dot/1(q_dot) -> chose which method/2

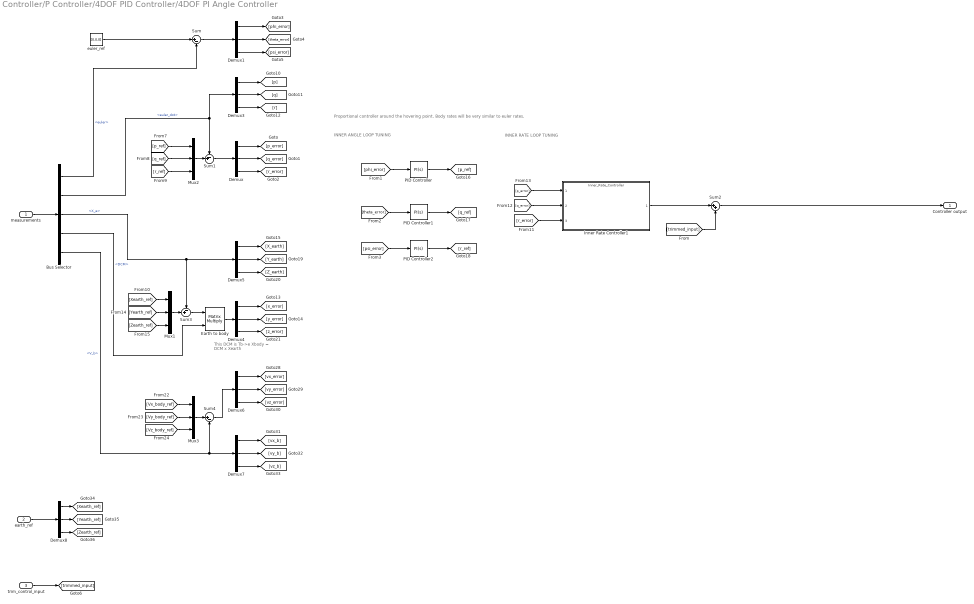
== system Controller/P Controller/4DOF PID Controller/4DOF PI Angle Controller ==
  note: This DCM is Tb->e
      | Xbody = DCM x Xearth
  note: Proportional controller around the hovering point. Body rates will be very similar to euler rates.
  note: INNER RATE LOOP TUNING
  note: INNER ANGLE LOOP TUNING
  measurements : Inport
  earth_ref : Inport  Port=2
  trim_control_input : Inport  Port=3
  Bus Selector : BusSelector  OutputSignals=euler,euler_dot,X_e,DCM,V_b
  Demux{,1,3..8} (8 alike) : Demux  Outputs=3
  Earth to body : Product  Multiplication=Matrix(*)
  Inner Rate Controller1 : ModelReference  ModelNameDialog=Inner_Rate_Controller  SimulationMode=Normal  ModelReferenceVersion=1.1241  CopyOfModelName=Inner_Rate_Controller
  Mux1 : Mux  Inputs=3
  Mux2 : Mux  Inputs=3
  Mux3 : Mux  Inputs=3
  PID Controller : simulink/Continuous/PID Controller  Controller=PI  TimeDomain=Continuous-time  SampleTime=-1  IntegratorMethod=Forward Euler  FilterMethod=Forward Euler  Form=Parallel  UseFilter=on  ControllerParametersSource=internal  P=1  I=1  D=0  N=100  InitialConditionSource=internal  InitialConditionForIntegrator=0  InitialConditionForFilter=0  ExternalReset=none  LimitOutput=off  UpperSaturationLimit=inf  LowerSaturationLimit=-inf  LinearizeAsGain=on  AntiWindupMode=none  Kb=1  TrackingMode=off  Kt=1  PParamMin=[]  PParamMax=[]  IParamMin=[]  IParamMax=[]  DParamMin=[]  DParamMax=[]  NParamMin=[]  NParamMax=[]  KbParamMin=[]  KbParamMax=[]  KtParamMin=[]  KtParamMax=[]  POutMin=[]  POutMax=[]  IOutMin=[]  IOutMax=[]  DOutMin=[]  DOutMax=[]  NOutMin=[]  NOutMax=[]  KbOutMin=[]  KbOutMax=[]  KtOutMin=[]  KtOutMax=[]  IntegratorOutMin=[]  IntegratorOutMax=[]  FilterOutMin=[]  FilterOutMax=[]  SumOutMin=[]  SumOutMax=[]  SumI1OutMin=[]  SumI1OutMax=[]  SumI2OutMin=[]  SumI2OutMax=[]  SumI3OutMin=[]  SumI3OutMax=[]  SumDOutMin=[]  SumDOutMax=[]  SaturationOutMin=[]  SaturationOutMax=[]  IntegratorContinuousStateAttributes=''  IntegratorStateMustResolveToSignalObject=off  IntegratorRTWStateStorageClass=Auto  FilterContinuousStateAttributes=''  FilterStateMustResolveToSignalObject=off  FilterRTWStateStorageClass=Auto  DifferentiatorICPrevScaledInput=0  DifferentiatorOutMin=[]  DifferentiatorOutMax=[]
  PID Controller1 : simulink/Continuous/PID Controller  Controller=PI  TimeDomain=Continuous-time  SampleTime=-1  IntegratorMethod=Forward Euler  FilterMethod=Forward Euler  Form=Parallel  UseFilter=on  ControllerParametersSource=internal  P=1  I=1  D=0  N=100  InitialConditionSource=internal  InitialConditionForIntegrator=0  InitialConditionForFilter=0  ExternalReset=none  LimitOutput=off  UpperSaturationLimit=inf  LowerSaturationLimit=-inf  LinearizeAsGain=on  AntiWindupMode=none  Kb=1  TrackingMode=off  Kt=1  PParamMin=[]  PParamMax=[]  IParamMin=[]  IParamMax=[]  DParamMin=[]  DParamMax=[]  NParamMin=[]  NParamMax=[]  KbParamMin=[]  KbParamMax=[]  KtParamMin=[]  KtParamMax=[]  POutMin=[]  POutMax=[]  IOutMin=[]  IOutMax=[]  DOutMin=[]  DOutMax=[]  NOutMin=[]  NOutMax=[]  KbOutMin=[]  KbOutMax=[]  KtOutMin=[]  KtOutMax=[]  IntegratorOutMin=[]  IntegratorOutMax=[]  FilterOutMin=[]  FilterOutMax=[]  SumOutMin=[]  SumOutMax=[]  SumI1OutMin=[]  SumI1OutMax=[]  SumI2OutMin=[]  SumI2OutMax=[]  SumI3OutMin=[]  SumI3OutMax=[]  SumDOutMin=[]  SumDOutMax=[]  SaturationOutMin=[]  SaturationOutMax=[]  IntegratorContinuousStateAttributes=''  IntegratorStateMustResolveToSignalObject=off  IntegratorRTWStateStorageClass=Auto  FilterContinuousStateAttributes=''  FilterStateMustResolveToSignalObject=off  FilterRTWStateStorageClass=Auto  DifferentiatorICPrevScaledInput=0  DifferentiatorOutMin=[]  DifferentiatorOutMax=[]
  PID Controller2 : simulink/Continuous/PID Controller  Controller=PI  TimeDomain=Continuous-time  SampleTime=-1  IntegratorMethod=Forward Euler  FilterMethod=Forward Euler  Form=Parallel  UseFilter=on  ControllerParametersSource=internal  P=1  I=0.1  D=0  N=100  InitialConditionSource=internal  InitialConditionForIntegrator=0  InitialConditionForFilter=0  ExternalReset=none  LimitOutput=off  UpperSaturationLimit=inf  LowerSaturationLimit=-inf  LinearizeAsGain=on  AntiWindupMode=none  Kb=1  TrackingMode=off  Kt=1  PParamMin=[]  PParamMax=[]  IParamMin=[]  IParamMax=[]  DParamMin=[]  DParamMax=[]  NParamMin=[]  NParamMax=[]  KbParamMin=[]  KbParamMax=[]  KtParamMin=[]  KtParamMax=[]  POutMin=[]  POutMax=[]  IOutMin=[]  IOutMax=[]  DOutMin=[]  DOutMax=[]  NOutMin=[]  NOutMax=[]  KbOutMin=[]  KbOutMax=[]  KtOutMin=[]  KtOutMax=[]  IntegratorOutMin=[]  IntegratorOutMax=[]  FilterOutMin=[]  FilterOutMax=[]  SumOutMin=[]  SumOutMax=[]  SumI1OutMin=[]  SumI1OutMax=[]  SumI2OutMin=[]  SumI2OutMax=[]  SumI3OutMin=[]  SumI3OutMax=[]  SumDOutMin=[]  SumDOutMax=[]  SaturationOutMin=[]  SaturationOutMax=[]  IntegratorContinuousStateAttributes=''  IntegratorStateMustResolveToSignalObject=off  IntegratorRTWStateStorageClass=Auto  FilterContinuousStateAttributes=''  FilterStateMustResolveToSignalObject=off  FilterRTWStateStorageClass=Auto  DifferentiatorICPrevScaledInput=0  DifferentiatorOutMin=[]  DifferentiatorOutMax=[]
  Sum : Sum  Inputs=|+-
  Sum1 : Sum  Inputs=-+|
  Sum2 : Sum  Inputs=|++
  Sum3 : Sum  Inputs=-+|
  Sum4 : Sum  Inputs=|+-
  euler_ref : Constant  Value=[0,0,0]
  Controller output : Outport
  wires:
  [psi_error] -> PID Controller2/1
  [theta_error] -> PID Controller1/1
  PID Controller2/1 -> [r_ref]
  PID Controller1/1 -> [q_ref]
  PID Controller/1 -> [p_ref]
  [phi_error] -> PID Controller/1
  Demux3/3 -> [r]
  Demux3/2 -> [q]
  Demux3/1 -> [p]
  measurements/1 -> Bus Selector/1
  Sum2/1 -> Controller output/1
  Bus Selector/2 -> Demux3/1, Sum1/1  "<euler_dot>"
  Sum1/1 -> Demux/1
  Demux/3 -> [r_error]
  Demux/2 -> [q_error]
  Demux/1 -> [p_error]
  trim_control_input/1 -> [trimmed_input]
  [trimmed_input] -> Sum2/2
  Mux2/1 -> Sum1/2
  [q_ref] -> Mux2/2
  [p_ref] -> Mux2/1
  [r_ref] -> Mux2/3
  Inner Rate Controller1/1 -> Sum2/1
  [p_error] -> Inner Rate Controller1/1
  [q_error] -> Inner Rate Controller1/2
  [r_error] -> Inner Rate Controller1/3
  Bus Selector/3 -> Demux5/1, Sum3/1  "<X_e>"
  Demux5/3 -> [Z_earth]
  Demux5/2 -> [Y_earth]
  Demux5/1 -> [X_earth]
  Demux4/3 -> [z_error]
  Demux4/2 -> [y_error]
  Demux4/1 -> [x_error]
  Mux1/1 -> Sum3/2
  [Yearth_ref] -> Mux1/2
  [Xearth_ref] -> Mux1/1
  [Zearth_ref] -> Mux1/3
  Mux3/1 -> Sum4/1
  Demux7/1 -> [vx_b]
  Demux7/2 -> [vy_b]
  Demux7/3 -> [vz_b]
  Bus Selector/5 -> Demux7/1, Sum4/2  "<V_b>"
  Sum4/1 -> Demux6/1
  Demux6/1 -> [vx_error]
  Demux6/2 -> [vy_error]
  Demux6/3 -> [vz_error]
  [Vy_body_ref] -> Mux3/2
  [Vx_body_ref] -> Mux3/1
  [Vz_body_ref] -> Mux3/3
  Bus Selector/4 -> Earth to body/2  "<DCM>"
  Earth to body/1 -> Demux4/1
  Sum3/1 -> Earth to body/1
  Demux8/3 -> [Zearth_ref]
  Demux8/2 -> [Yearth_ref]
  Demux8/1 -> [Xearth_ref]
  earth_ref/1 -> Demux8/1
  Bus Selector/1 -> Sum/2  "<euler>"
  Sum/1 -> Demux1/1
  Demux1/1 -> [phi_error]
  Demux1/2 -> [theta_error]
  Demux1/3 -> [psi_error]
  euler_ref/1 -> Sum/1
